simulink model "SM1"  (R2024a)
settings: Solver=VariableStepAuto  StartTime=0.0  StopTime=10.0  RelTol=1e-3
values from neighbouring files (symbols this model uses):
  A_m = (n_m * K_t * n_g * K_g)/R_m    (= 0.33398001)    [sm1.m]
  B_eq = 1    [sm1.m]
  J_eq = 0.0017728    [sm1.m]
  K_bb = 5 / 7 * (g * r_arm) / L_plaque    (= 0.41838605682)    [sm1.m]
libraries: simulink x1
settings Model: Creator=lfgon  LastModifiedBy=lfgon
settings DataIOCC: ReturnWorkspaceOutputs=off

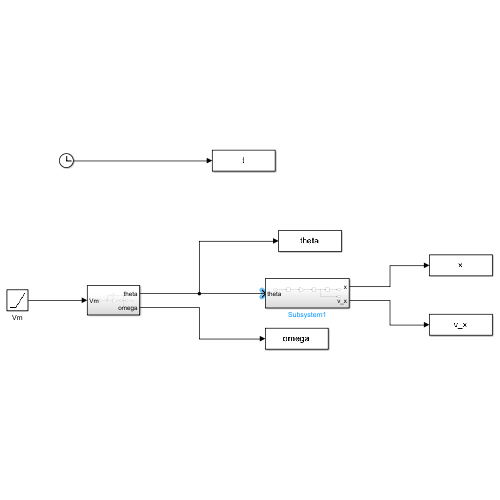
[thumbnail: Simulink's stored preview of the top-level diagram]
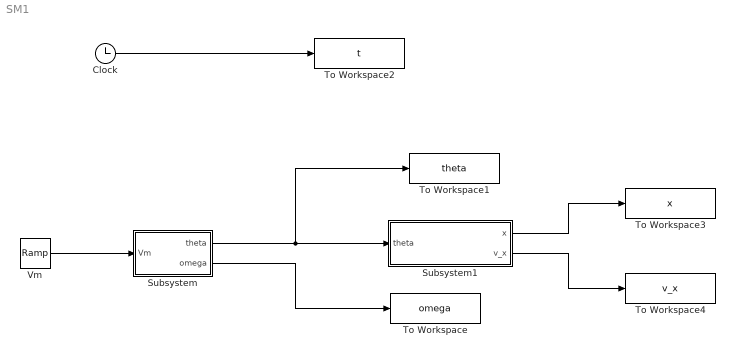
== system SM1 ==
  Clock : Clock
  Subsystem : Subsystem
  Subsystem1 : Subsystem
  To Workspace : ToWorkspace  VariableName=omega  SampleTime=-1
  To Workspace1 : ToWorkspace  VariableName=theta  SampleTime=-1
  To Workspace2 : ToWorkspace  VariableName=t  SampleTime=-1
  To Workspace3 : ToWorkspace  VariableName=x  SampleTime=-1
  To Workspace4 : ToWorkspace  VariableName=v_x  SampleTime=-1
  Vm : simulink/Sources/Ramp  slope=1  start=0  InitialOutput=0
  wires:
  Clock/1 -> To Workspace2/1
  Vm/1 -> Subsystem/1(Vm)
  Subsystem/2(omega) -> To Workspace/1
  Subsystem/1(theta) -> To Workspace1/1, Subsystem1/1(theta)
  Subsystem1/1(x) -> To Workspace3/1
  Subsystem1/2(v_x) -> To Workspace4/1

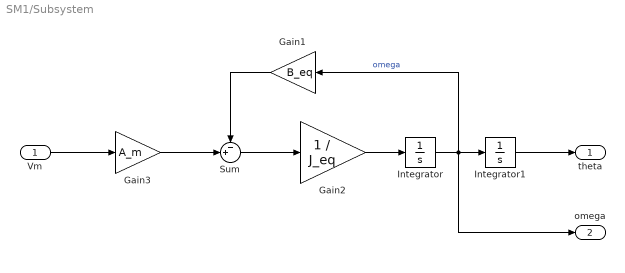
== system SM1/Subsystem ==
  Vm : Inport
  Gain1 : Gain  Gain=B_eq
  Gain2 : Gain  Gain=1 / J_eq
  Gain3 : Gain  Gain=A_m
  Integrator : Integrator
  Integrator1 : Integrator
  Sum : Sum  Inputs=-+|
  theta : Outport
  omega : Outport  Port=2
  wires:
  Sum/1 -> Gain2/1
  Vm/1 -> Gain3/1
  Integrator/1 -> omega/1, Gain1/1, Integrator1/1  "omega"
  Gain1/1 -> Sum/1
  Gain3/1 -> Sum/2
  Gain2/1 -> Integrator/1
  Integrator1/1 -> theta/1

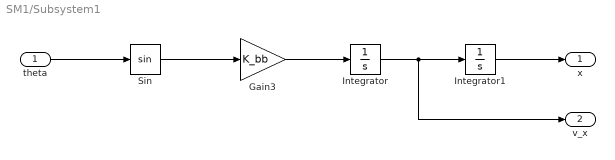
== system SM1/Subsystem1 ==
  theta : Inport
  Gain3 : Gain  Gain=K_bb
  Integrator : Integrator
  Integrator1 : Integrator
  Sin : Trigonometry
  x : Outport
  v_x : Outport  Port=2
  wires:
  Integrator/1 -> v_x/1, Integrator1/1
  Gain3/1 -> Integrator/1
  Integrator1/1 -> x/1
  theta/1 -> Sin/1
  Sin/1 -> Gain3/1
